simulink model "SVPWM_SPWM_180_120"  (R2020b)
settings: Solver=ode23s  StartTime=0.0  StopTime=0.15  FixedStep=1e-6  MaxStep=1e-6  RelTol=1e-4
undefined symbols (not defined in the file): Tperiod
libraries: powerlib x20, simulink x2, powerlib_meascontrol x2
settings Model: Creator=User  LastModifiedBy=ahmed
settings DataIOCC: ReturnWorkspaceOutputs=off

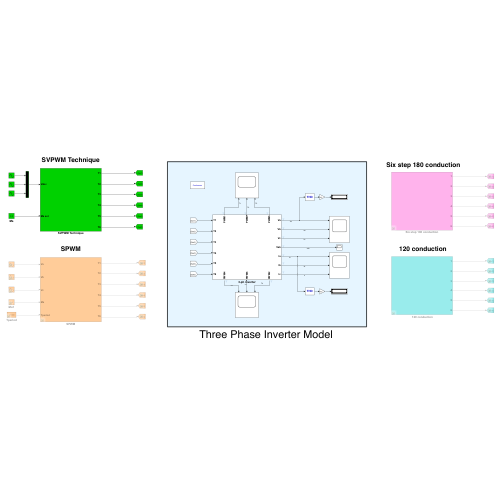
[thumbnail: Simulink's stored preview of the top-level diagram]
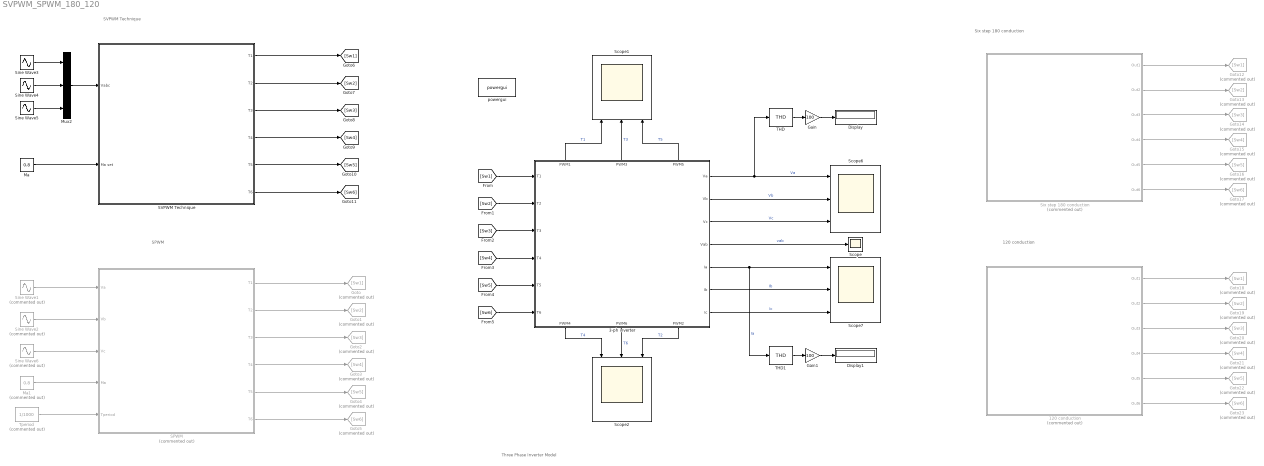
== system SVPWM_SPWM_180_120 ==
  note: SVPWM Technique
  note: Three Phase Inverter Model
  note: SPWM
  note: Six step 180 conduction
  note: 120 conduction
  " 120 conduction" : Subsystem  Commented=on
  3-ph inverter : Subsystem
      settings: PortSchema="{\"entries\":[{\"content\":{\"sides\":[{\"content\":{\"connectorIds\":[\"In1\",\"In2\",\"In3\",\"In4\",\"In5\",\"In6\"]},\"type\":\"ConnectorPlacement.EquallySpacedRectSide\",\"uuid\":\"9670f19d-de72-4ce0-97fc-2d99c77c4947\"},{\"content\":{\"connectorIds\":[\"Out1\",\"Out2\",\"Out3\",\"Out4\",\"Out5\",\"Out6\",\"Out7\"],\"side\":\"RIGHT\"},\"type\":\"ConnectorPlacement.EquallySpacedRectSide\",\"uuid\":\"898fb6ae-88ba-4ea3-b291-10dfcbbe4f4c\"},{\"content\":{\"connectorIds\":[\"Out11\",\"Out12\",\"Out13\"],\"side\":\"TOP\"},\"type\":\"ConnectorPlacement.EquallySpacedRectSide\",\"uuid\":\"97eb4227-aa82-44c6-9db4-9e2937822b7b\"},{\"content\":{\"connectorIds\":[\"Out8\",\"Out9\",\"Out10\"],\"side\":\"BOTTOM\"},\"type\":\"ConnectorPlacement.EquallySpacedRectSide\",\"uuid\":\"00673fcf-d9a4-45b1-91ba-2ca0356fde6c\"}]},\"type\":\"ConnectorPlacement.EquallySpacedConnector\",\"uuid\":\"520770ab-a4b7-4c47-9972-ee71a59cf9a8\"}],\"packageUris\":[\"http://schema.mathworks.com/mf0/Connector/R2020b\"],\"version\":\"1.0\"}"
  Display : Display
  Display1 : Display
  Gain : Gain  Gain=100
  Gain1 : Gain  Gain=100
  Goto : Goto  Commented=on  GotoTag=Sw1
  Goto1 : Goto  Commented=on  GotoTag=Sw2
  Goto12 : Goto  Commented=on  GotoTag=Sw1
  Goto13 : Goto  Commented=on  GotoTag=Sw2
  Goto14 : Goto  Commented=on  GotoTag=Sw3
  Goto15 : Goto  Commented=on  GotoTag=Sw4
  Goto16 : Goto  Commented=on  GotoTag=Sw5
  Goto17 : Goto  Commented=on  GotoTag=Sw6
  Goto18 : Goto  Commented=on  GotoTag=Sw1
  Goto19 : Goto  Commented=on  GotoTag=Sw2
  Goto2 : Goto  Commented=on  GotoTag=Sw3
  Goto20 : Goto  Commented=on  GotoTag=Sw3
  Goto21 : Goto  Commented=on  GotoTag=Sw4
  Goto22 : Goto  Commented=on  GotoTag=Sw5
  Goto23 : Goto  Commented=on  GotoTag=Sw6
  Goto3 : Goto  Commented=on  GotoTag=Sw4
  Goto4 : Goto  Commented=on  GotoTag=Sw5
  Goto5 : Goto  Commented=on  GotoTag=Sw6
  Ma : Constant  Value=0.8
  Ma1 : Constant  Commented=on  Value=0.8
  Mux2 : Mux  Inputs=3
  SPWM : Subsystem  Commented=on
  SVPWM Technique : Subsystem
  Scope : Scope
  Scope{1..2,6..7} (4 alike) : Scope  NumInputPorts=3
  Sine Wave1 : Sin  Commented=on  Amplitude=0.8  Frequency=2*pi*50  SampleTime=0
  Sine Wave2 : Sin  Commented=on  Amplitude=0.8  Frequency=2*pi*50  Phase=-2*pi/3  SampleTime=0
  Sine Wave3 : Sin  Amplitude=100*0.8*1/sqrt(3)  Frequency=2*pi*50  SampleTime=0
  Sine Wave4 : Sin  Amplitude=100*0.8*1/sqrt(3)  Frequency=2*pi*50  Phase=-2*pi/3  SampleTime=0
  Sine Wave5 : Sin  Amplitude=100*0.8*1/sqrt(3)  Frequency=2*pi*50  Phase=2*pi/3  SampleTime=0
  Sine Wave6 : Sin  Commented=on  Amplitude=0.8  Frequency=2*pi*50  Phase=2*pi/3  SampleTime=0
  Six step 180 conduction : Subsystem  Commented=on
  THD : powerlib_meascontrol/Measurements/THD  Freq=50  Ts=0
  THD1 : powerlib_meascontrol/Measurements/THD  Freq=50  Ts=0
  Tperiod : Constant  Commented=on  Value=1/1000
  powergui : powerlib/powergui  Priority=1  SimulationMode=Continuous  SampleTime=50e-6  frequency=60  Iterations=50  frequencyindice=0  Pbase=100e6  ErrMax=1e-4  UnitsV=kV  UnitsW=MW  buscounter=0  FunctionMessages=off  echomessages=off  EnableUseOfTLC=off  CurrentSourceSwitches=off  DisableSnubberDevices=off  DisableRonSwitches=off  DisableVfSwitches=off  DisplayEquations=off  AutomaticDiscreteSolvers=off  SolverType=Tustin/Backward Euler (TBE)  Interpol=off  ExternalGateDelay=off  methode=off  Ts=100  x0status=blocks  SPID=on  SwTol=0  HookPort=off  NonlinearTolerance=1e-4  nMaxIteration=100  ContinueOnMaxIteration=off  RestoreLinks=warning  ResistiveCurrentMeasurement=off  Frange=[0:2:500]  Ylog=off  Xlog=on  ShowGrid=off  save=off  variable=ZData  structure=0  ZoomFFT=off  StartTime=0.0  cycles=1  DisplayStyle=1  fundamental=60  FreqAxis=off  MaxFrequency=1000  frequencyindicesteady=1  RmsSteady=1  display=off
  wires:
  3-ph inverter/5(Ia) -> Scope7/1, THD1/1  "Ia"
  3-ph inverter/11(PWM1) -> Scope1/1  "T1"
  3-ph inverter/7(Ic) -> Scope7/3  "Ic"
  3-ph inverter/4(Vab) -> Scope/1  "vab"
  3-ph inverter/13(PWM5) -> Scope1/3  "T5"
  3-ph inverter/6(Ib) -> Scope7/2  "Ib"
  3-ph inverter/2(Vb) -> Scope6/2  "Vb"
  3-ph inverter/1(Va) -> Scope6/1, THD/1  "Va"
  3-ph inverter/3(Vc) -> Scope6/3  "Vc"
  Mux2/1 -> SVPWM Technique/1(Vabc)
  Sine Wave4/1 -> Mux2/2
  Sine Wave5/1 -> Mux2/3
  Sine Wave3/1 -> Mux2/1
  Ma/1 -> SVPWM Technique/2(Ma set)
  Sine Wave1/1 -> SPWM/1(Va)
  Sine Wave6/1 -> SPWM/3(Vc)
  Sine Wave2/1 -> SPWM/2(Vb)
  Ma1/1 -> SPWM/4(Ma)
  Tperiod/1 -> SPWM/5(Tperiod)
  [Sw1] -> 3-ph inverter/1(T1)
  [Sw2] -> 3-ph inverter/2(T2)
  [Sw3] -> 3-ph inverter/3(T3)
  [Sw4] -> 3-ph inverter/4(T4)
  [Sw5] -> 3-ph inverter/5(T5)
  [Sw6] -> 3-ph inverter/6(T6)
  SPWM/5(T5) -> Goto4/1
  SPWM/4(T4) -> Goto3/1
  SPWM/3(T3) -> Goto2/1
  SPWM/6(T6) -> Goto5/1
  SPWM/2(T2) -> Goto1/1
  SPWM/1(T1) -> Goto/1
  SVPWM Technique/1(T1) -> [Sw1]
  SVPWM Technique/2(T2) -> [Sw2]
  SVPWM Technique/3(T3) -> [Sw3]
  SVPWM Technique/4(T4) -> [Sw4]
  SVPWM Technique/5(T5) -> [Sw5]
  SVPWM Technique/6(T6) -> [Sw6]
  Six step 180 conduction/4(Out4) -> Goto15/1
  Six step 180 conduction/3(Out3) -> Goto14/1
  Six step 180 conduction/5(Out5) -> Goto16/1
  Six step 180 conduction/2(Out2) -> Goto13/1
  Six step 180 conduction/6(Out6) -> Goto17/1
  Six step 180 conduction/1(Out1) -> Goto12/1
  " 120 conduction"/1(Out1) -> Goto18/1
  " 120 conduction"/6(Out6) -> Goto23/1
  " 120 conduction"/2(Out2) -> Goto19/1
  " 120 conduction"/5(Out5) -> Goto22/1
  " 120 conduction"/3(Out3) -> Goto20/1
  " 120 conduction"/4(Out4) -> Goto21/1
  3-ph inverter/12(PWM3) -> Scope1/2  "T3"
  THD/1 -> Gain/1
  Gain/1 -> Display/1
  THD1/1 -> Gain1/1
  Gain1/1 -> Display1/1
  3-ph inverter/8(PWM4) -> Scope2/1  "T4"
  3-ph inverter/9(PWM6) -> Scope2/2  "T6"
  3-ph inverter/10(PWM2) -> Scope2/3  "T2"

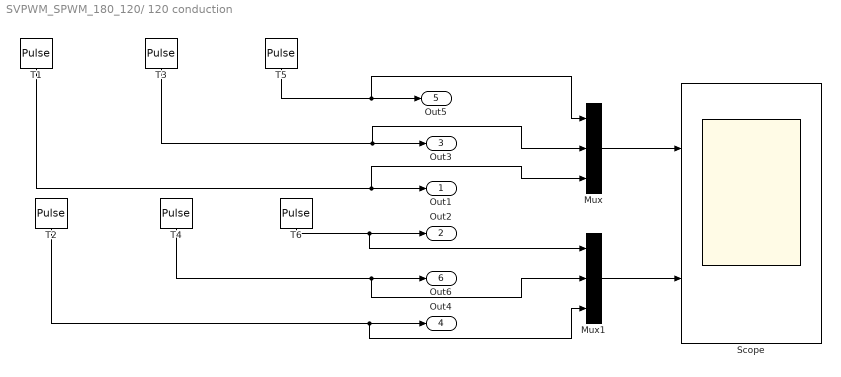
== system SVPWM_SPWM_180_120/ 120 conduction ==
  Mux : Mux  Inputs=3
  Mux1 : Mux  Inputs=3
  Scope : Scope  NumInputPorts=2
  T1 : DiscretePulseGenerator  PulseType=Time based  Period=Tperiod  PulseWidth=30
  T2 : DiscretePulseGenerator  PulseType=Time based  Period=Tperiod  PulseWidth=30  PhaseDelay=Tperiod/2
  T3 : DiscretePulseGenerator  PulseType=Time based  Period=Tperiod  PulseWidth=30  PhaseDelay=Tperiod/3
  T4 : DiscretePulseGenerator  PulseType=Time based  Period=Tperiod  PulseWidth=30  PhaseDelay=5*Tperiod/6
  T5 : DiscretePulseGenerator  PulseType=Time based  Period=Tperiod  PulseWidth=30  PhaseDelay=2*Tperiod/3
  T6 : DiscretePulseGenerator  PulseType=Time based  Period=Tperiod  PulseWidth=30  PhaseDelay=7*Tperiod/6
  Out1 : Outport
  Out2 : Outport  Port=2
  Out3 : Outport  Port=3
  Out4 : Outport  Port=4
  Out5 : Outport  Port=5
  Out6 : Outport  Port=6
  wires:
  T5/1 -> Mux/1, Out5/1
  T3/1 -> Mux/2, Out3/1
  T1/1 -> Mux/3, Out1/1
  T2/1 -> Mux1/3, Out4/1
  T4/1 -> Mux1/2, Out6/1
  T6/1 -> Mux1/1, Out2/1
  Mux/1 -> Scope/1
  Mux1/1 -> Scope/2

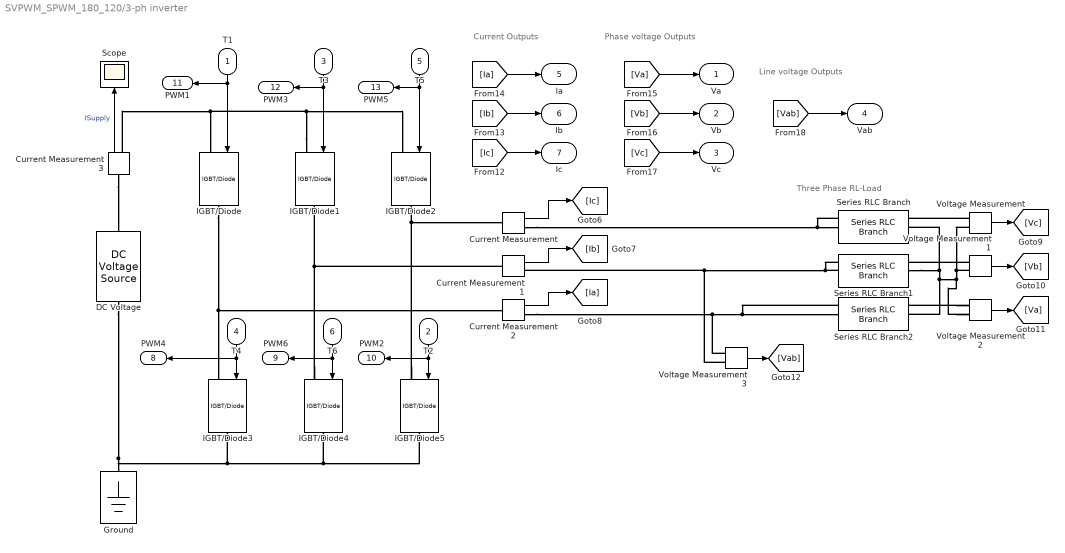
== system SVPWM_SPWM_180_120/3-ph inverter ==
  note: Current Outputs
  note: Phase voltage Outputs
  note: Line voltage Outputs
  note: Three Phase RL-Load
  T1 : Inport
  T2 : Inport  Port=2
  T3 : Inport  Port=3
  T4 : Inport  Port=4
  T5 : Inport  Port=5
  T6 : Inport  Port=6
  Current Measurement{,1..3} (4 alike) : powerlib/Measurements/Current Measurement  PhasorSimulation=off  OutputType=Complex  PSBequivalent=0
  DC Voltage : powerlib/Electrical Sources/DC Voltage Source  Amplitude=100  Measurements=None
  Ground : powerlib/Elements/Ground  LConnTagsString=a
  IGBT/Diode{,1..5} (6 alike) : powerlib/Power Electronics/IGBT//Diode  Ron=1e-3  Rs=1e5  Cs=inf  Measurements=off
  Scope : Scope
  Series RLC Branch : powerlib/Elements/Series RLC Branch  LConnTagsString=__new0  RConnTagsString=__new0  BranchType=RL  Resistance=1  Inductance=5e-3  SetiL0=off  InitialCurrent=0  Capacitance=1e-6  Setx0=off  InitialVoltage=0  Measurements=None
  Series RLC Branch1 : powerlib/Elements/Series RLC Branch  LConnTagsString=__new0  RConnTagsString=__new0  BranchType=RL  Resistance=1  Inductance=5e-3  SetiL0=off  InitialCurrent=0  Capacitance=1e-6  Setx0=off  InitialVoltage=0  Measurements=None
  Series RLC Branch2 : powerlib/Elements/Series RLC Branch  LConnTagsString=__new0  RConnTagsString=__new0  BranchType=RL  Resistance=1  Inductance=5e-3  SetiL0=off  InitialCurrent=0  Capacitance=1e-6  Setx0=off  InitialVoltage=0  Measurements=None
  Voltage Measurement{,1..3} (4 alike) : powerlib/Measurements/Voltage Measurement  PhasorSimulation=off  OutputType=Complex  PSBequivalent=0
  Va : Outport
  Vb : Outport  Port=2
  Vc : Outport  Port=3
  Vab : Outport  Port=4
  Ia : Outport  Port=5
  Ib : Outport  Port=6
  Ic : Outport  Port=7
  PWM4 : Outport  Port=8
  PWM6 : Outport  Port=9
  PWM2 : Outport  Port=10
  PWM1 : Outport  Port=11
  PWM3 : Outport  Port=12
  PWM5 : Outport  Port=13
  wires:
  T3/1 -> IGBT/Diode1/1, PWM3/1
  Voltage Measurement3/1 -> [Vab]
  Current Measurement2/1 -> [Ia]
  T4/1 -> IGBT/Diode3/1, PWM4/1
  T5/1 -> IGBT/Diode2/1, PWM5/1
  T1/1 -> IGBT/Diode/1, PWM1/1
  T6/1 -> IGBT/Diode4/1, PWM6/1
  Current Measurement1/1 -> [Ib]
  [Vb] -> Vb/1
  Voltage Measurement2/1 -> [Va]
  T2/1 -> IGBT/Diode5/1, PWM2/1
  [Vc] -> Vc/1
  [Va] -> Va/1
  Current Measurement/1 -> [Ic]
  Voltage Measurement/1 -> [Vc]
  Voltage Measurement1/1 -> [Vb]
  [Vab] -> Vab/1
  [Ia] -> Ia/1
  [Ib] -> Ib/1
  [Ic] -> Ic/1
  Current Measurement3/1 -> Scope/1  "ISupply"
  connections:
  Voltage Measurement/LConn2 -- Series RLC Branch1/RConn1 -- Series RLC Branch/RConn1 -- Series RLC Branch2/RConn1 -- Voltage Measurement2/LConn2 -- Voltage Measurement1/LConn2
  Voltage Measurement2/LConn1 -- Current Measurement2/RConn1 -- Voltage Measurement3/LConn1 -- Series RLC Branch2/LConn1
  IGBT/Diode1/LConn1 -- Current Measurement3/RConn1 -- IGBT/Diode/LConn1 -- IGBT/Diode2/LConn1
  IGBT/Diode5/RConn1 -- IGBT/Diode4/RConn1 -- DC Voltage/LConn1 -- Ground/LConn1 -- IGBT/Diode3/RConn1
  Series RLC Branch1/LConn1 -- Voltage Measurement3/LConn2 -- Current Measurement1/RConn1 -- Voltage Measurement1/LConn1
  Current Measurement/RConn1 -- Series RLC Branch/LConn1 -- Voltage Measurement/LConn1
  IGBT/Diode4/LConn1 -- IGBT/Diode1/RConn1 -- Current Measurement1/LConn1
  IGBT/Diode5/LConn1 -- Current Measurement/LConn1 -- IGBT/Diode2/RConn1
  IGBT/Diode/RConn1 -- Current Measurement2/LConn1 -- IGBT/Diode3/LConn1
  Current Measurement3/LConn1 -- DC Voltage/RConn1

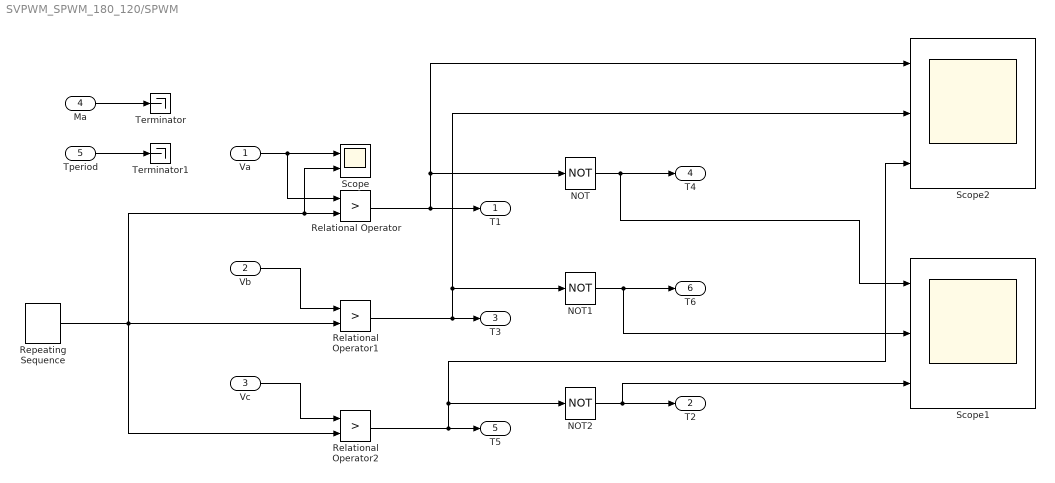
== system SVPWM_SPWM_180_120/SPWM ==
  Va : Inport
  Vb : Inport  Port=2
  Vc : Inport  Port=3
  Ma : Inport  Port=4
  Tperiod : Inport  Port=5
  NOT : Logic  Operator=NOT  IconShape=distinctive  AllPortsSameDT=off  OutDataTypeStr=boolean
  NOT1 : Logic  Operator=NOT  IconShape=distinctive  AllPortsSameDT=off  OutDataTypeStr=boolean
  NOT2 : Logic  Operator=NOT  IconShape=distinctive  AllPortsSameDT=off  OutDataTypeStr=boolean
  Relational Operator : RelationalOperator  Operator=>  OutDataTypeStr=boolean  RndMeth=Simplest
  Relational Operator1 : RelationalOperator  Operator=>  OutDataTypeStr=boolean  RndMeth=Simplest
  Relational Operator2 : RelationalOperator  Operator=>  OutDataTypeStr=boolean  RndMeth=Simplest
  Repeating Sequence : simulink/Sources/Repeating Sequence  rep_seq_t="[ 0  (1/15000)/4  (1/15000)/2  3*(1/15000)/4  (1/15000) ]"  rep_seq_y=[ 0 1 0 -1 0 ]
  Scope : Scope  NumInputPorts=2
  Scope1 : Scope  NumInputPorts=3
  Scope2 : Scope  NumInputPorts=3
  Terminator : Terminator
  Terminator1 : Terminator
  T1 : Outport
  T2 : Outport  Port=2
  T3 : Outport  Port=3
  T4 : Outport  Port=4
  T5 : Outport  Port=5
  T6 : Outport  Port=6
  wires:
  Va/1 -> Relational Operator/1, Scope/1
  Repeating Sequence/1 -> Scope/2, Relational Operator/2, Relational Operator2/2, Relational Operator1/2
  Vb/1 -> Relational Operator1/1
  Vc/1 -> Relational Operator2/1
  Relational Operator/1 -> T1/1, NOT/1, Scope2/1
  Relational Operator1/1 -> Scope2/2, NOT1/1, T3/1
  Relational Operator2/1 -> NOT2/1, Scope2/3, T5/1
  NOT/1 -> Scope1/1, T4/1
  NOT1/1 -> Scope1/2, T6/1
  NOT2/1 -> Scope1/3, T2/1
  Ma/1 -> Terminator/1
  Tperiod/1 -> Terminator1/1

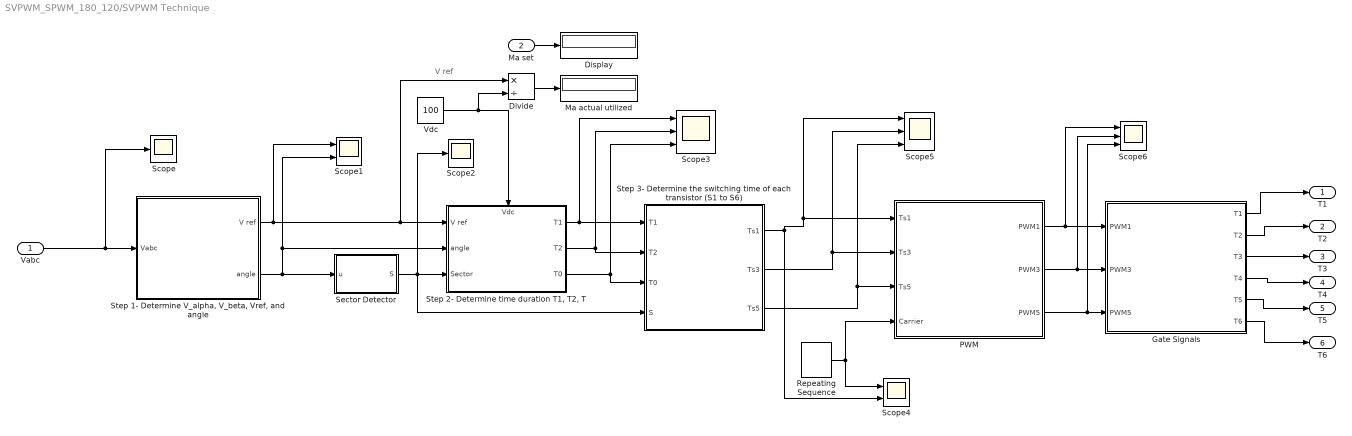
== system SVPWM_SPWM_180_120/SVPWM Technique ==
  note: V ref
  Vabc : Inport
  Ma set : Inport  Port=2
  Display : Display
  Divide : Product  Inputs=*/
  Gate Signals : Subsystem
  Ma actual utilized : Display
  PWM : Subsystem
  Repeating Sequence : simulink/Sources/Repeating Sequence  rep_seq_t=[ 0 1/30000 1/15000 ]  rep_seq_y=[ 0 1/15000 0 ]
  Scope : Scope
  Scope1 : Scope  NumInputPorts=2
  Scope2 : Scope
  Scope3 : Scope  NumInputPorts=3
  Scope4 : Scope  NumInputPorts=2
  Scope5 : Scope  NumInputPorts=3
  Scope6 : Scope  NumInputPorts=3
  Sector Detector : MATLAB Function  TreatAsAtomicUnit=on
  "Step 1- Determine V_alpha, V_beta, Vref, and angle" : Subsystem
  "Step 2- Determine time duration T1, T2, T" : Subsystem
      settings: PortSchema="{\"entries\":[{\"content\":{\"sides\":[{\"content\":{\"connectorIds\":[\"In1\",\"In2\",\"In3\"]},\"type\":\"ConnectorPlacement.EquallySpacedRectSide\",\"uuid\":\"2dad9b71-fb55-40e3-9250-08671b06fd76\"},{\"content\":{\"connectorIds\":[\"Out1\",\"Out2\",\"Out3\"],\"side\":\"RIGHT\"},\"type\":\"ConnectorPlacement.EquallySpacedRectSide\",\"uuid\":\"fd9577f6-2035-4946-b366-efd909fd578d\"},{\"content\":{\"connectorIds\":[\"In4\"],\"side\":\"TOP\"},\"type\":\"ConnectorPlacement.EquallySpacedRectSide\",\"uuid\":\"03f93542-188d-4be0-9359-187a882052ac\"}]},\"type\":\"ConnectorPlacement.EquallySpacedConnector\",\"uuid\":\"0cec5607-3333-48e6-b527-ee7f13af7673\"}],\"packageUris\":[\"http://schema.mathworks.com/mf0/Connector/R2020b\"],\"version\":\"1.0\"}"
  "Step 3- Determine the switching time of each transistor (S1 to S6) " : Subsystem
  Vdc : Constant  Value=100
  T1 : Outport
  T2 : Outport  Port=2
  T3 : Outport  Port=3
  T4 : Outport  Port=4
  T5 : Outport  Port=5
  T6 : Outport  Port=6
  wires:
  Repeating Sequence/1 -> Scope4/1, PWM/4(Carrier)
  "Step 2- Determine time duration T1, T2, T"/3(T0) -> Scope3/3, "Step 3- Determine the switching time of each transistor (S1 to S6) "/3(T0)
  "Step 1- Determine V_alpha, V_beta, Vref, and angle"/2(angle) -> Scope1/2, "Step 2- Determine time duration T1, T2, T"/2(angle), Sector Detector/1(u)
  PWM/2(PWM3) -> Scope6/2, Gate Signals/2(PWM3)
  Gate Signals/4(T4) -> T4/1
  Sector Detector/1(S) -> "Step 3- Determine the switching time of each transistor (S1 to S6) "/4(S), Scope2/1, "Step 2- Determine time duration T1, T2, T"/3(Sector)
  Vdc/1 -> Divide/2, "Step 2- Determine time duration T1, T2, T"/4(Vdc)
  Gate Signals/2(T2) -> T2/1
  "Step 2- Determine time duration T1, T2, T"/1(T1) -> Scope3/1, "Step 3- Determine the switching time of each transistor (S1 to S6) "/1(T1)
  PWM/1(PWM1) -> Scope6/1, Gate Signals/1(PWM1)
  "Step 2- Determine time duration T1, T2, T"/2(T2) -> Scope3/2, "Step 3- Determine the switching time of each transistor (S1 to S6) "/2(T2)
  Vabc/1 -> Scope/1, "Step 1- Determine V_alpha, V_beta, Vref, and angle"/1(Vabc)
  Divide/1 -> Ma actual utilized/1
  PWM/3(PWM5) -> Scope6/3, Gate Signals/3(PWM5)
  Gate Signals/6(T6) -> T6/1
  "Step 3- Determine the switching time of each transistor (S1 to S6) "/1(Ts1) -> Scope5/1, PWM/1(Ts1), Scope4/2
  "Step 3- Determine the switching time of each transistor (S1 to S6) "/2(Ts3) -> Scope5/2, PWM/2(Ts3)
  "Step 3- Determine the switching time of each transistor (S1 to S6) "/3(Ts5) -> Scope5/3, PWM/3(Ts5)
  Gate Signals/5(T5) -> T5/1
  Gate Signals/1(T1) -> T1/1
  Gate Signals/3(T3) -> T3/1
  "Step 1- Determine V_alpha, V_beta, Vref, and angle"/1(V ref) -> Scope1/1, Divide/1, "Step 2- Determine time duration T1, T2, T"/1(V ref)
  Ma set/1 -> Display/1

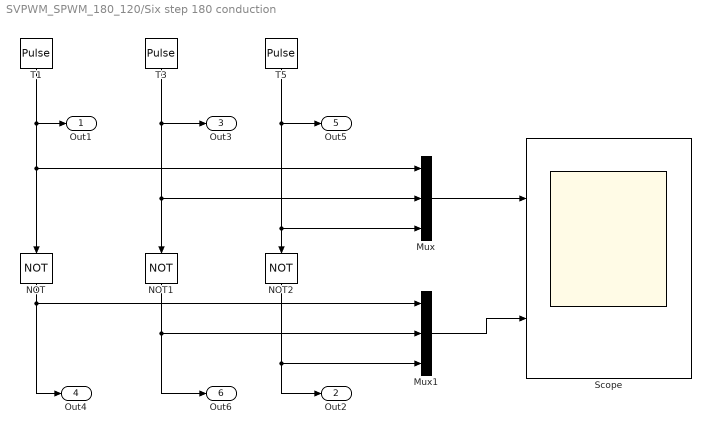
== system SVPWM_SPWM_180_120/Six step 180 conduction ==
  Mux : Mux  Inputs=3
  Mux1 : Mux  Inputs=3
  NOT : Logic  Operator=NOT  IconShape=distinctive  AllPortsSameDT=off  OutDataTypeStr=boolean
  NOT1 : Logic  Operator=NOT  IconShape=distinctive  AllPortsSameDT=off  OutDataTypeStr=boolean
  NOT2 : Logic  Operator=NOT  IconShape=distinctive  AllPortsSameDT=off  OutDataTypeStr=boolean
  Scope : Scope  NumInputPorts=2
  T1 : DiscretePulseGenerator  PulseType=Time based  Period=20e-3  PulseWidth=50
  T3 : DiscretePulseGenerator  PulseType=Time based  Period=20e-3  PulseWidth=50  PhaseDelay=((20e-3)/3)
  T5 : DiscretePulseGenerator  PulseType=Time based  Period=20e-3  PulseWidth=50  PhaseDelay=(2*(20e-3)/3)
  Out1 : Outport
  Out2 : Outport  Port=2
  Out3 : Outport  Port=3
  Out4 : Outport  Port=4
  Out5 : Outport  Port=5
  Out6 : Outport  Port=6
  wires:
  T1/1 -> NOT/1, Mux/1, Out1/1
  T3/1 -> Mux/2, NOT1/1, Out3/1
  T5/1 -> Mux/3, NOT2/1, Out5/1
  NOT/1 -> Mux1/1, Out4/1
  NOT1/1 -> Mux1/2, Out6/1
  Mux1/1 -> Scope/2
  Mux/1 -> Scope/1
  NOT2/1 -> Mux1/3, Out2/1

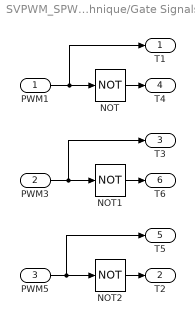
== system SVPWM_SPWM_180_120/SVPWM Technique/Gate Signals ==
  PWM1 : Inport
  PWM3 : Inport  Port=2
  PWM5 : Inport  Port=3
  NOT : Logic  Operator=NOT  IconShape=distinctive  AllPortsSameDT=off  OutDataTypeStr=boolean
  NOT1 : Logic  Operator=NOT  IconShape=distinctive  AllPortsSameDT=off  OutDataTypeStr=boolean
  NOT2 : Logic  Operator=NOT  IconShape=distinctive  AllPortsSameDT=off  OutDataTypeStr=boolean
  T1 : Outport
  T2 : Outport  Port=2
  T3 : Outport  Port=3
  T4 : Outport  Port=4
  T5 : Outport  Port=5
  T6 : Outport  Port=6
  wires:
  PWM1/1 -> T1/1, NOT/1
  NOT/1 -> T4/1
  NOT1/1 -> T6/1
  PWM3/1 -> T3/1, NOT1/1
  PWM5/1 -> T5/1, NOT2/1
  NOT2/1 -> T2/1

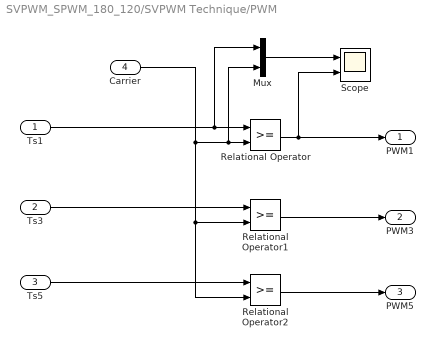
== system SVPWM_SPWM_180_120/SVPWM Technique/PWM ==
  Ts1 : Inport
  Ts3 : Inport  Port=2
  Ts5 : Inport  Port=3
  Carrier : Inport  Port=4
  Mux : Mux  Inputs=2
  Relational Operator : RelationalOperator  OutDataTypeStr=boolean  RndMeth=Simplest
  Relational Operator1 : RelationalOperator  OutDataTypeStr=boolean  RndMeth=Simplest
  Relational Operator2 : RelationalOperator  OutDataTypeStr=boolean  RndMeth=Simplest
  Scope : Scope  NumInputPorts=2
  PWM1 : Outport
  PWM3 : Outport  Port=2
  PWM5 : Outport  Port=3
  wires:
  Ts1/1 -> Mux/1, Relational Operator/1
  Ts3/1 -> Relational Operator1/1
  Ts5/1 -> Relational Operator2/1
  Carrier/1 -> Relational Operator2/2, Relational Operator1/2, Mux/2, Relational Operator/2
  Relational Operator/1 -> Scope/2, PWM1/1
  Relational Operator1/1 -> PWM3/1
  Relational Operator2/1 -> PWM5/1
  Mux/1 -> Scope/1

== system SVPWM_SPWM_180_120/SVPWM Technique/Step 1- Determine V_alpha, V_beta, Vref, and angle ==
  Vabc : Inport
  Demux : Demux  Outputs=3
  Polar form : Subsystem
  "Power invariant Clark transformation " : Subsystem
  Scope : Scope  NumInputPorts=2
  V ref : Outport
  angle : Outport  Port=2
  wires:
  Vabc/1 -> Demux/1
  Demux/2 -> "Power invariant Clark transformation "/2(Vb)
  Demux/1 -> "Power invariant Clark transformation "/1(Va)
  Demux/3 -> "Power invariant Clark transformation "/3(Vc)
  "Power invariant Clark transformation "/1(V alpha) -> Scope/1, Polar form/1(In1)
  "Power invariant Clark transformation "/2(V beta) -> Scope/2, Polar form/2(In2)
  Polar form/1(V ref) -> V ref/1
  Polar form/2(angle) -> angle/1

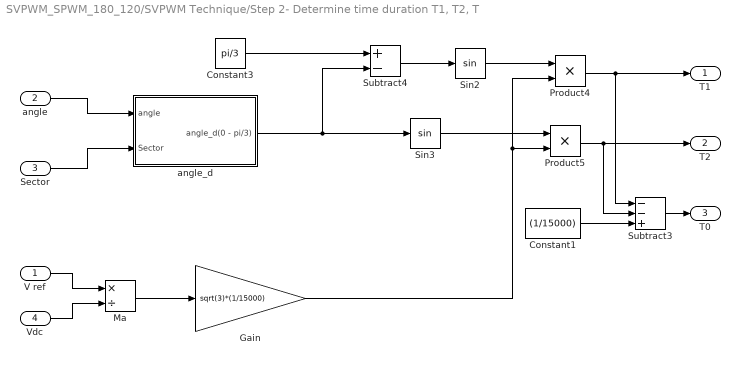
== system SVPWM_SPWM_180_120/SVPWM Technique/Step 2- Determine time duration T1, T2, T ==
  V ref : Inport
  angle : Inport  Port=2
  Sector : Inport  Port=3
  Vdc : Inport  Port=4
  Constant1 : Constant  Value=(1/15000)
  Constant3 : Constant  Value=pi/3
  Gain : Gain  Gain=sqrt(3)*(1/15000)
  Ma : Product  Inputs=*/
  Product4 : Product
  Product5 : Product
  Sin2 : Trigonometry
  Sin3 : Trigonometry
  Subtract3 : Sum  Inputs=--+
  Subtract4 : Sum  Inputs=+-
  angle_d : Subsystem
  T1 : Outport
  T2 : Outport  Port=2
  T0 : Outport  Port=3
  wires:
  angle/1 -> angle_d/1(angle)
  Sector/1 -> angle_d/2(Sector)
  V ref/1 -> Ma/1
  Vdc/1 -> Ma/2
  Constant3/1 -> Subtract4/1
  angle_d/1(angle_d(0 - pi/3)) -> Sin3/1, Subtract4/2
  Subtract4/1 -> Sin2/1
  Ma/1 -> Gain/1
  Sin2/1 -> Product4/1
  Gain/1 -> Product4/2, Product5/2
  Product4/1 -> Subtract3/1, T1/1
  Sin3/1 -> Product5/1
  Product5/1 -> Subtract3/2, T2/1
  Subtract3/1 -> T0/1
  Constant1/1 -> Subtract3/3

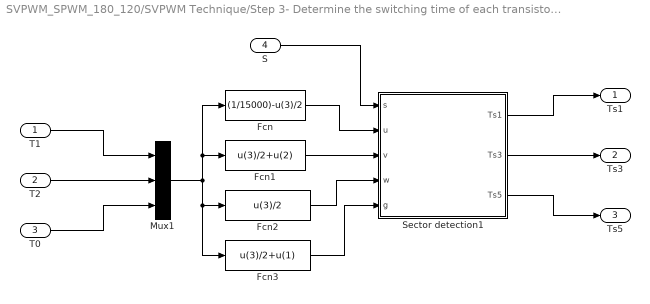
== system SVPWM_SPWM_180_120/SVPWM Technique/Step 3- Determine the switching time of each transistor (S1 to S6)  ==
  T1 : Inport
  T2 : Inport  Port=2
  T0 : Inport  Port=3
  S : Inport  Port=4
  Fcn : Fcn  Expr=(1/15000)-u(3)/2
  Fcn1 : Fcn  Expr=u(3)/2+u(2)
  Fcn2 : Fcn  Expr=u(3)/2
  Fcn3 : Fcn  Expr=u(3)/2+u(1)
  Mux1 : Mux  Inputs=3
  Sector detection1 : MATLAB Function  TreatAsAtomicUnit=on
  Ts1 : Outport
  Ts3 : Outport  Port=2
  Ts5 : Outport  Port=3
  wires:
  S/1 -> Sector detection1/1(s)
  Fcn1/1 -> Sector detection1/3(v)
  Mux1/1 -> Fcn/1, Fcn1/1, Fcn3/1, Fcn2/1
  Fcn3/1 -> Sector detection1/5(g)
  Fcn/1 -> Sector detection1/2(u)
  Fcn2/1 -> Sector detection1/4(w)
  T1/1 -> Mux1/1
  T2/1 -> Mux1/2
  T0/1 -> Mux1/3
  Sector detection1/2(Ts3) -> Ts3/1
  Sector detection1/3(Ts5) -> Ts5/1
  Sector detection1/1(Ts1) -> Ts1/1

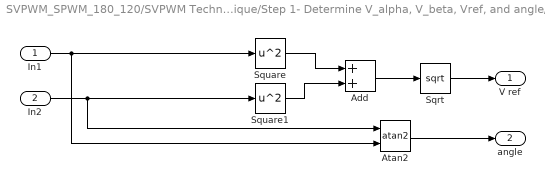
== system SVPWM_SPWM_180_120/SVPWM Technique/Step 1- Determine V_alpha, V_beta, Vref, and angle/Polar form ==
  In1 : Inport
  In2 : Inport  Port=2
  Add : Sum
  Atan2 : Trigonometry  Operator=atan2
  Sqrt : Sqrt  SaturateOnIntegerOverflow=on
  Square : Math  Operator=square  SaturateOnIntegerOverflow=on
  Square1 : Math  Operator=square  SaturateOnIntegerOverflow=on
  V ref : Outport
  angle : Outport  Port=2
  wires:
  Square1/1 -> Add/2
  Square/1 -> Add/1
  Atan2/1 -> angle/1
  In2/1 -> Atan2/1, Square1/1
  Sqrt/1 -> V ref/1
  Add/1 -> Sqrt/1
  In1/1 -> Atan2/2, Square/1

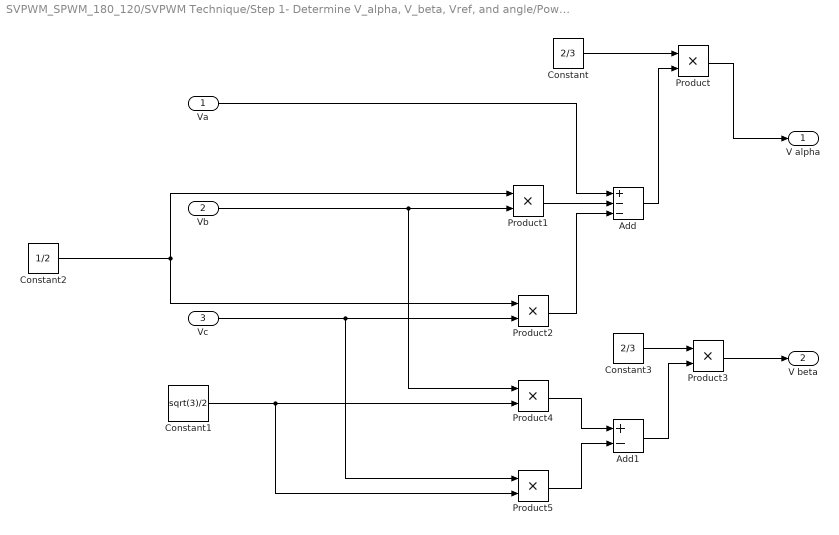
== system SVPWM_SPWM_180_120/SVPWM Technique/Step 1- Determine V_alpha, V_beta, Vref, and angle/Power invariant Clark transformation  ==
  Va : Inport
  Vb : Inport  Port=2
  Vc : Inport  Port=3
  Add : Sum  Inputs=+--
  Add1 : Sum  Inputs=+-
  Constant : Constant  Value=2/3
  Constant1 : Constant  Value=sqrt(3)/2
  Constant2 : Constant  Value=1/2
  Constant3 : Constant  Value=2/3
  Product{,1..5} (6 alike) : Product
  V alpha : Outport
  V beta : Outport  Port=2
  wires:
  Product/1 -> V alpha/1
  Product3/1 -> V beta/1
  Constant/1 -> Product/1
  Va/1 -> Add/1
  Vb/1 -> Product1/2, Product4/1
  Product1/1 -> Add/2
  Product2/1 -> Add/3
  Vc/1 -> Product2/2, Product5/1
  Constant2/1 -> Product2/1, Product1/1
  Add/1 -> Product/2
  Constant3/1 -> Product3/1
  Add1/1 -> Product3/2
  Constant1/1 -> Product5/2, Product4/2
  Product4/1 -> Add1/1
  Product5/1 -> Add1/2

== system SVPWM_SPWM_180_120/SVPWM Technique/Step 2- Determine time duration T1, T2, T/angle_d ==
  angle : Inport
  Sector : Inport  Port=2
  Constant3 : Constant
  Gain : Gain  Gain=pi/3
  Subtract4 : Sum  Inputs=-+
  Subtract5 : Sum  Inputs=+-
  angle_d(0 - pi/3) : Outport
  wires:
  angle/1 -> Subtract4/2
  Sector/1 -> Subtract5/1
  Subtract4/1 -> angle_d(0 - pi/3)/1
  Constant3/1 -> Subtract5/2
  Subtract5/1 -> Gain/1
  Gain/1 -> Subtract4/1

== matlab function SVPWM_SPWM_180_120/SVPWM Technique/Sector Detector ==
  data: u input; S output
function S = fcn(u)

  u= 180/(pi)*u ; % rad to degree
  
if (u>=0)&&(u<60)
  u = 1  ; 
elseif (u>=60)&&(u<120)
  u = 2  ;  
elseif (u>=120)&&(u<180)
  u = 3  ;  
elseif (u>=-180)&&(u<-120)
  u = 4  ;
elseif (u>=-120)&&(u<-60)
  u = 5  ;
elseif (u>=-60)&&(u<0)
  u = 6  ;
else
  u=0 ; 
end

S = u;

== matlab function SVPWM_SPWM_180_120/SVPWM Technique/Step 3- Determine the switching time of each transistor (S1 to S6) /Sector detection1 ==
  data: s input; u input; Ts1 output; Ts3 output; v input; w input; g input; Ts5 output
function [Ts1,Ts3,Ts5] = fcn(s,u,v,w,g)

switch s 
  
 case 1 
  Ts1 = u ; 
  Ts3 = v ;
  Ts5 = w ;
 case 2 
  Ts1 = g ; 
  Ts3 = u ; 
  Ts5 = w ;
 case 3 
  Ts1 = w ;
  Ts3 = u ; 
  Ts5 = v ; 
 case 4 
  Ts1 = w ;
  Ts3 = g ; 
  Ts5 = u ;
 case 5 
  Ts1 = v ;
  Ts3 = w ; 
  Ts5 = u ;
 case 6 
  Ts1 = u ;
  Ts3 = w ; 
  Ts5 = g ;
 otherwise 
  Ts1 = 0 ; 
 Ts3 = 0 ;
 Ts5 = 0 ;
 end 

end
